simulink library "m3dof_library"  (Simulink 7.6)
settings: Solver=ode45  StartTime=0.0  StopTime=10.0  RelTol=1e-3
values from neighbouring files (symbols this model uses):
  eg = [0 1 0]    [init.m]
  I1 = 4/12*m1*l1^2    (= 0.111111111111)    [init.m]
  I2 = 4/12*m2*l2^2    (= 0.111111111111)    [init.m]
  I3 = 4/12*m3*l3^2    (= 0.111111111111)    [init.m]
  l1 = 1/3    (= 0.333333333333)    [init.m]
  l2 = 1/3    (= 0.333333333333)    [init.m]
  l3 = 1/3    (= 0.333333333333)    [init.m]
  m1 = 3    [init.m]
  m2 = 3    [init.m]
  m3 = 3    [init.m]
  mx1 = m1*l1/2    (= 0.5)    [init.m]
  mx2 = m2*l2/2    (= 0.5)    [init.m]
  mx3 = m3*l3/2    (= 0.5)    [init.m]
settings Model: Creator=Gmalex  LastModifiedBy=Gmalex

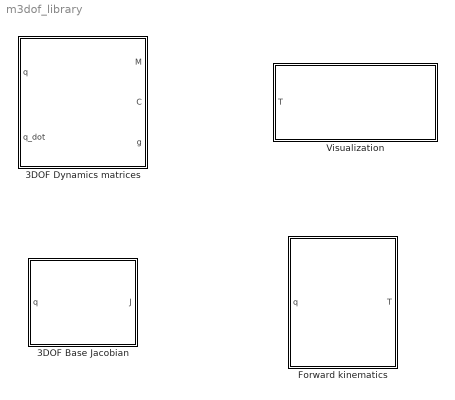
== system m3dof_library ==
  3DOF Base Jacobian : Subsystem  AncestorBlock=library/Forward kinematics  mask{a1=l1, a2=l2, a3=l3}
      mask prompts: a1 "Linklength (Link 1)"; a2 "Linklength (Link 2)"; a3 "Linklength (Link 3)"
      mask help: Base Jacobian of a the 3DoF Manipulator.
  3DOF Dynamics matrices : Subsystem  mask(Dynamics matrices){m1=m1, mX1=mx1, ZZ1=I1, m2=m2, mX2=mx2, ZZ2=I2, m3=m3, mX3=mx3, ZZ3=I3, a1=l1, a2=l2, a3=l3, eg=eg}
      mask prompts: m1 "Mass (Link1)"; mX1 "Massmoment 1. Order (Link1)"; ZZ1 "Massmoment 2. Order (Link 1)"; m2 "Mass (Link2)"; mX2 "Massmoment 1. Order (Link2)"; ZZ2 "Massmoment 2. Order (Link2)"; m3 "Mass (Link3)"; mX3 "Massmoment 1. Order (Link3)"; ZZ3 "Massmoment 2. Order (Link3)"; a1 "Link lenght (Link 1)"; a2 "Link lenght (Link 2)"; a3 "Link lenght (Link 3)"; eg "Gravity direction"
      mask help:
      | Dynamics matrices of the planar 3 Dof manipulator, with q, qdot and eg
      | as joint position, joint velocity and unit vector pointing in (opposite)
      | direction of gravity. The Outputs are M (3x3), C (3x3) and G (3x1) as
      | mass matrix, coriolis and centrifugal matrix and gravity vector.
  Forward kinematics : Subsystem  mask{a1=l1, a2=l2, a3=l3, alpha=0}
      mask prompts: a1 "Linklength (Link 1)"; a2 "Linklength (Link 2)"; a3 "Linklength (Link 3)"; alpha "TCP Orientation"
      mask help:
      | Forward kinematics of the 3DOF planarmanipulator.
      | - q: joint angles
      | - T: bus containing the homogeneous transformation matrices for each link
  Visualization : Subsystem  mask{Ts0=1/16, al=1, a1=l1, a2=l2, a3=l3, alpha=0, eg=eg, tl=50}
      mask prompts: Ts0 "Sample Time Animation"; al "Plot Axis Limit"; a1 "Linklength (Link 1)"; a2 "Linklength (Link 2)"; a3 "Linklength (Link 3)"; alpha "TCP Orientation"; eg "Unitvector (Oposite Gravity direction)"; tl "Tracelength"
      mask help:
      | Visualization utility for the 3DOF planar manipulator.
      | - T: bus containing the homogeneous transformation matrices for each link

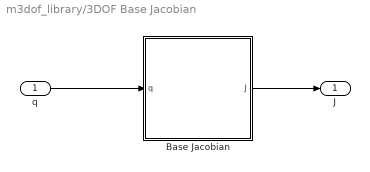
== system m3dof_library/3DOF Base Jacobian ==
  q : Inport
  Base Jacobian : Stateflow chart  TreatAsAtomicUnit=on
  J : Outport
  wires:
  q/1 -> Base Jacobian/1(q)
  Base Jacobian/1(J) -> J/1

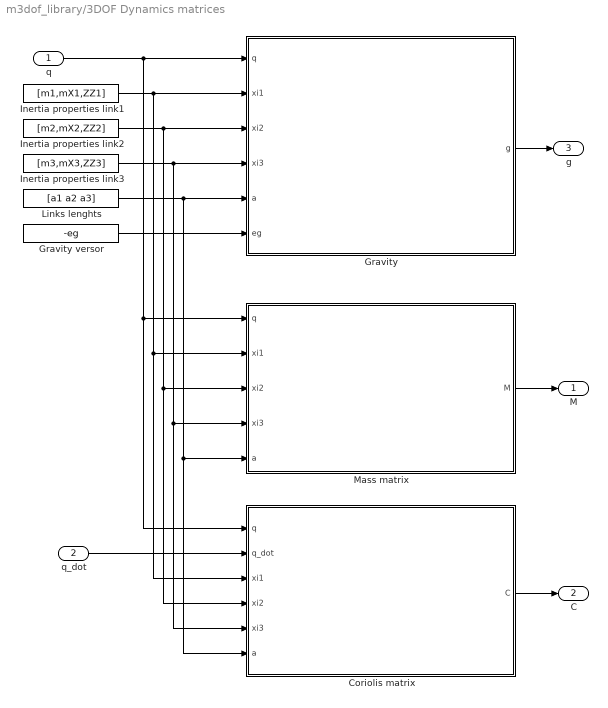
== system m3dof_library/3DOF Dynamics matrices ==
  q : Inport
  q_dot : Inport  Port=2
  Coriolis matrix : Stateflow chart  TreatAsAtomicUnit=on
  Gravity : Stateflow chart  TreatAsAtomicUnit=on
  Gravity versor : Constant  Value=-eg
  Inertia properties link1 : Constant  Value=[m1,mX1,ZZ1]
  Inertia properties link2 : Constant  Value=[m2,mX2,ZZ2]
  Inertia properties link3 : Constant  Value=[m3,mX3,ZZ3]
  Links lenghts : Constant  Value=[a1 a2 a3]
  Mass matrix : Stateflow chart  TreatAsAtomicUnit=on
  M : Outport
  C : Outport  Port=2
  g : Outport  Port=3
  wires:
  q/1 -> Gravity/1(q), Mass matrix/1(q), Coriolis matrix/1(q)
  Gravity/1(g) -> g/1
  Inertia properties link1/1 -> Gravity/2(xi1), Mass matrix/2(xi1), Coriolis matrix/3(xi1)
  Inertia properties link2/1 -> Gravity/3(xi2), Mass matrix/3(xi2), Coriolis matrix/4(xi2)
  Inertia properties link3/1 -> Gravity/4(xi3), Mass matrix/4(xi3), Coriolis matrix/5(xi3)
  Links lenghts/1 -> Gravity/5(a), Mass matrix/5(a), Coriolis matrix/6(a)
  Gravity versor/1 -> Gravity/6(eg)
  Mass matrix/1(M) -> M/1
  Coriolis matrix/1(C) -> C/1
  q_dot/1 -> Coriolis matrix/2(q_dot)

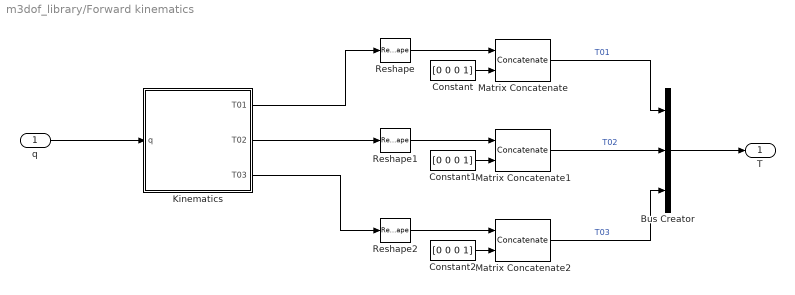
== system m3dof_library/Forward kinematics ==
  q : Inport
  Bus Creator : BusCreator  Inputs=3
  Constant : Constant  Value=[0 0 0 1]  VectorParams1D=off
  Constant1 : Constant  Value=[0 0 0 1]  VectorParams1D=off
  Constant2 : Constant  Value=[0 0 0 1]  VectorParams1D=off
  Kinematics : Stateflow chart  TreatAsAtomicUnit=on
  Matrix Concatenate : Concatenate  Mode=Multidimensional array
  Matrix Concatenate1 : Concatenate  Mode=Multidimensional array
  Matrix Concatenate2 : Concatenate  Mode=Multidimensional array
  Reshape : Reshape  OutputDimensionality=Customize  OutputDimensions=[3,4]
  Reshape1 : Reshape  OutputDimensionality=Customize  OutputDimensions=[3,4]
  Reshape2 : Reshape  OutputDimensionality=Customize  OutputDimensions=[3,4]
  T : Outport
  wires:
  Kinematics/1(T01) -> Reshape/1
  q/1 -> Kinematics/1(q)
  Kinematics/3(T03) -> Reshape2/1
  Kinematics/2(T02) -> Reshape1/1
  Reshape/1 -> Matrix Concatenate/1
  Constant/1 -> Matrix Concatenate/2
  Matrix Concatenate/1 -> Bus Creator/1  "T01"
  Reshape1/1 -> Matrix Concatenate1/1
  Constant1/1 -> Matrix Concatenate1/2
  Constant2/1 -> Matrix Concatenate2/2
  Reshape2/1 -> Matrix Concatenate2/1
  Matrix Concatenate1/1 -> Bus Creator/2  "T02"
  Matrix Concatenate2/1 -> Bus Creator/3  "T03"
  Bus Creator/1 -> T/1

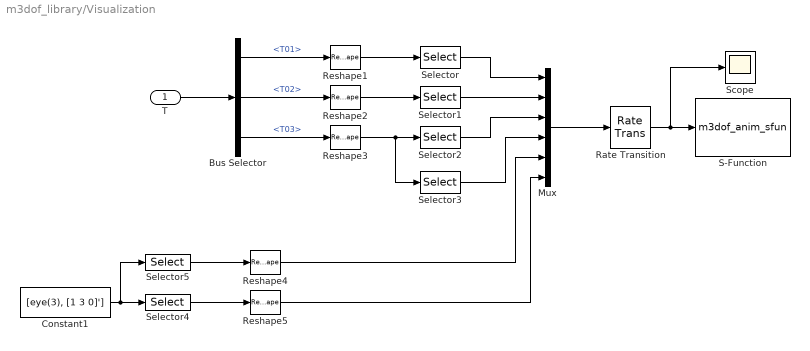
== system m3dof_library/Visualization ==
  T : Inport
  Bus Selector : BusSelector  OutputSignals=T01,T02,T03
  Constant1 : Constant  Value=[eye(3), [1 3 0]']
  Mux : Mux  Inputs=6
  Rate Transition : RateTransition  OutPortSampleTime=Ts0
  Reshape{1..5} (5 alike) : Reshape
  S-Function : S-Function  FunctionName=m3dof_anim_sfun  Parameters=Ts0,al,eg,tl  EnableBusSupport=off
  Scope : Scope
  Selector : Selector  InputPortWidth=16  IndexOptions=Index vector (dialog)  Indices=[13 14]  OutputSizes=1
  Selector1 : Selector  InputPortWidth=16  IndexOptions=Index vector (dialog)  Indices=[13 14]  OutputSizes=1
  Selector2 : Selector  InputPortWidth=16  IndexOptions=Index vector (dialog)  Indices=[13 14]  OutputSizes=1
  Selector3 : Selector  InputPortWidth=16  IndexOptions=Index vector (dialog)  Indices=[1 2 5 6]  OutputSizes=1
  Selector4 : Selector  NumberOfDimensions=2  InputPortWidth=3  IndexOptions=Index vector (dialog),Index vector (dialog)  Indices=1:2,1:2  OutputSizes=1,1
  Selector5 : Selector  NumberOfDimensions=2  InputPortWidth=3  IndexOptions=Index vector (dialog),Index vector (dialog)  Indices=1:2,4  OutputSizes=1,1
  wires:
  Reshape1/1 -> Selector/1
  Reshape2/1 -> Selector1/1
  Reshape3/1 -> Selector2/1, Selector3/1
  Mux/1 -> Rate Transition/1
  Selector/1 -> Mux/1
  Selector1/1 -> Mux/2
  Selector2/1 -> Mux/3
  Rate Transition/1 -> S-Function/1, Scope/1
  Selector3/1 -> Mux/4
  Bus Selector/1 -> Reshape1/1  "<T01>"
  Bus Selector/3 -> Reshape3/1  "<T03>"
  Constant1/1 -> Selector4/1, Selector5/1
  Selector5/1 -> Reshape4/1
  Reshape4/1 -> Mux/5
  Selector4/1 -> Reshape5/1
  Reshape5/1 -> Mux/6
  T/1 -> Bus Selector/1
  Bus Selector/2 -> Reshape2/1  "<T02>"

== matlab function Forward kinematics/Kinematics ==
  data: q input double; T01 output double; T02 output double; T03 output double; l1 parameter double; l2 parameter double; l3 parameter double
function [T01,T02,T03] = fcn(q, l1, l2, l3)
%#eml

% Angles calculation
c1 = cos(q(1));
s1 = sin(q(1));
c12 = cos(q(1) + q(2));
s12 = sin(q(1) + q(2));
c123 = cos(q(1) + q(2) + q(3));
s123 = sin(q(1) + q(2) + q(3));

% Homogeneous matrices
T01 = [c1 -s1 0 l1*c1; s1 c1 0 l1*s1; 0 0 1 0];
T02 = [c12 -s12 0 (l1*c1 + l2*c12); s12 c12 0 (l1*s1 + l2*s12); 0 0 1 0];
T03 = [c123 -s123 0 (l1*c1 + l2*c12 + l3*c123); s123 c123 0 (l1*s1 + l2*s12 + l3*s123); 0 0 1 0];

== matlab function 3DOF Dynamics matrices/Coriolis matrix ==
  data: q input double size=3; q_dot input double; xi1 input double size=3; C output double; xi2 input double size=3; xi3 input double size=3; a input double size=3
function C = fcn(q, q_dot,xi1, xi2, xi3, a)

% Declaration and costants
C = zeros(3,3);
CORIOLIS = zeros(3,3);


% Support variables
qp = q_dot;
t1 = cos(q(3));
t2 = sin(q(2));
t3 = t1 * t2;
t5 = qp(2) * a(1) * xi3(2);
t6 = t3 * t5;
t7 = sin(q(3));
t8 = cos(q(2));
t9 = t7 * t8;
t11 = qp(3) * a(1) * xi3(2);
t12 = t9 * t11;
t13 = t3 * t11;
t14 = t2 * qp(2);
t16 = a(1) * a(2) * xi3(1);
t17 = t14 * t16;
t19 = a(2) * xi3(2);
t20 = t7 * qp(3) * t19;
t21 = t9 * t5;
t22 = a(1) * xi2(2);
t23 = t14 * t22;
t25 = qp(1) * a(1);
t26 = t25 * xi3(2);
t27 = t9 * t26;
t28 = t2 * qp(1);
t29 = t28 * t22;
t30 = t28 * t16;
t31 = t3 * t26;
t32 = -t13 - t27 - t29 - t6 - t12 - t21 - t30 - t17 - t31 - t23 - t20;
t33 = qp(1) + qp(2) + qp(3);
CORIOLIS(1,1) = -t6 - t12 - t13 - t17 - t20 - t21 - t23;
CORIOLIS(1,2) = t32;
CORIOLIS(1,3) = -t33 * (t3 * a(1) + t7 * a(2) + t9 * a(1)) * xi3(2);
CORIOLIS(2,1) = t31 + t29 - t20 + t30 + t27;
CORIOLIS(2,2) = -t20;
CORIOLIS(2,3) = -t7 * t33 * t19;
CORIOLIS(3,1) = (t9 * t25 + t3 * t25 + t7 * qp(2) * a(2) + t7 * qp(1) * a(2)) * xi3(2);
CORIOLIS(3,2) = t7 * (qp(1) + qp(2)) * t19;
CORIOLIS(3,3) = 0.0e0;



% Inertia matrix
for i = 1:3
    for j = 1:3
        C(i,j) = CORIOLIS(j,i);
    end
end

end

== matlab function 3DOF Dynamics matrices/Gravity ==
  data: q input double size=3; xi1 input double size=3; g output double; xi2 input double size=3; xi3 input double size=3; a input double size=3; eg input double
function g = fcn(q, xi1, xi2, xi3, a, eg)

%g0 = 9.81;

% Data extraction
%m1 = link1_mi(1);
%m2 = link2_mi(1);
%m3 = link2_mi(1);

% Angles calculation
%c1 = cos(q(1));
%s1 = sin(q(1));
%c12 = cos(q(1) + q(2));
%s12 = sin(q(1) + q(2));
%c123 = cos(q(1) + q(2) + q(3));
%s123 = sin(q(1) + q(2) + q(3));

% Gravity calculation
%g(1) = -()

g = zeros(3,1);

g0 = -9.81;



t1 = sin(q(1));
t2 = eg(1) * t1;
t4 = cos(q(1));
t5 = eg(1) * t4;
t6 = sin(q(2));
t7 = t6 * xi2(2);
t8 = t5 * t7;
t9 = cos(q(2));
t10 = t9 * xi2(2);
t11 = t2 * t10;
t12 = eg(2) * t1;
t13 = t12 * t7;
t14 = eg(2) * t4;
t15 = t14 * t10;
t16 = a(1) * xi2(1);
t19 = a(1) * xi3(1);
t22 = sin(q(3));
t23 = eg(1) * t22;
t24 = t1 * t6;
t25 = t24 * xi3(2);
t26 = t23 * t25;
t27 = cos(q(3));
t28 = eg(1) * t27;
t29 = t4 * t6;
t30 = t29 * xi3(2);
t31 = t28 * t30;
t32 = t2 * xi1(2) + t8 + t11 + t13 - t15 - t14 * t16 + t2 * t16 - t14 * t19 + t2 * t19 - t26 + t31;
t33 = t1 * t9;
t34 = t33 * xi3(2);
t35 = t28 * t34;
t37 = t9 * a(2) * xi3(1);
t38 = t2 * t37;
t39 = eg(2) * t22;
t40 = t39 * t30;
t42 = t6 * a(2) * xi3(1);
t43 = t12 * t42;
t44 = eg(2) * t27;
t45 = t4 * t9;
t46 = t45 * xi3(2);
t47 = t44 * t46;
t48 = t39 * t34;
t49 = t5 * t42;
t50 = t44 * t25;
t51 = t14 * t37;
t53 = t23 * t46;
t54 = t35 + t38 + t40 + t43 - t47 + t48 + t49 + t50 - t51 - t14 * xi1(2) + t53;
t57 = t53 - t26 + t50 + t8 + t13 + t35 + t49 - t15 + t40 + t48 + t11 - t51 - t47 + t43 + t38 + t31;
g(1) = -g0 * (t32 + t54);
g(2) = -g0 * t57;
g(3) = -g0 * (t28 * t29 + t28 * t33 + t23 * t45 - t23 * t24 - t44 * t45 + t44 * t24 + t39 * t29 + t39 * t33) * xi3(2);

end

== matlab function 3DOF Dynamics matrices/Mass matrix ==
  data: q input double size=3; xi1 input double size=3; M output double; xi2 input double size=3; xi3 input double size=3; a input double size=3
function M = fcn(q, xi1, xi2, xi3, a)

% Declaration and costants
M = zeros(3,3);
MAS = zeros(3,3);

% Support variables
t1 = a(1)^2;
t3 = cos(q(3));
t4 = cos(q(2));
t6 = a(1) * xi3(2);
t7 = t3 * t4 * t6;
t9 = sin(q(3));
t10 = sin(q(2));
t12 = t9 * t10 * t6;
t14 = a(2)^2;
t15 = t14 * xi3(1);
t16 = t4 * a(1);
t18 = t16 * a(2) * xi3(1);
t20 = t16 * xi2(2);
t23 = t3 * a(2) * xi3(2);
t24 = 0.2e1 * t23;
t26 = xi3(3) + t1 * xi2(1) + 0.2e1 * t7 - 0.2e1 * t12 + xi2(3) + xi1(3) + t15 + 0.2e1 * t18 + 0.2e1 * t20 + t24 + t1 * xi3(1);
t27 = xi2(3) + t20 + t15 + t18 - t12 + t24 + xi3(3) + t7;
t28 = xi3(3) - t12 + t7 + t23;
t30 = xi3(3) + t23;
MAS(1,1) = t26;
MAS(1,2) = t27;
MAS(1,3) = t28;
MAS(2,1) = t27;
MAS(2,2) = xi3(3) + xi2(3) + t24 + t15;
MAS(2,3) = t30;
MAS(3,1) = t28;
MAS(3,2) = t30;
MAS(3,3) = xi3(3);


% Inertia matrix
for i = 1:3
    for j = 1:3
        M(i,j) = MAS(j,i);
    end
end

end

== matlab function 3DOF Base Jacobian/Base Jacobian ==
  data: q input double; J output double; l1 parameter double; l2 parameter double; l3 parameter double
function J  = fcn(q, l1, l2, l3)
% Declaration
J = zeros(3,3);

% Angles calculation
c1 = cos(q(1));
s1 = sin(q(1));
c12 = cos(q(1) + q(2));
s12 = sin(q(1) + q(2));
c123 = cos(q(1) + q(2) + q(3));
s123 = sin(q(1) + q(2) + q(3));

% Jacobian calculation
J(1,1) = -l1*s1 -l2*s12 -l3*s123;
J(1,2) = -l2*s12 -l3*s123;
J(1,3) = -l3*s123;
J(2,1) = l1*c1 + l2*c12 + l3*c123;
J(2,2) = l2*c12 + l3*c123;
J(2,3) = l3*c123;
J(3,1) = 1;
J(3,2) = 1;
J(3,3) = 1;
